simulink model "smd_closedloop"  (R2026a)
settings: Solver=VariableStepAuto  StopTime=12
undefined symbols (not defined in the file): c, k, m
settings Model: Creator=tdxt  LastModifiedBy=tdxt

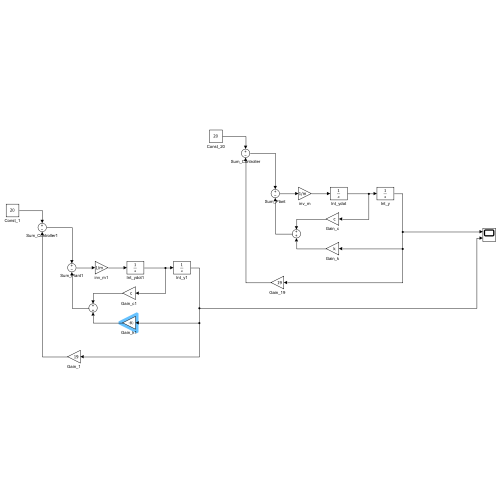
[thumbnail: Simulink's stored preview of the top-level diagram]
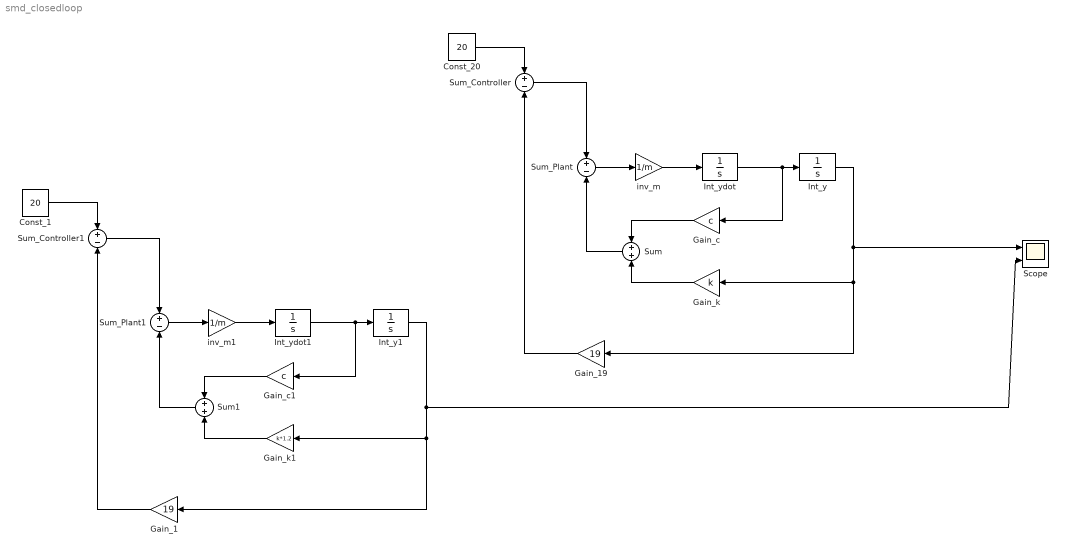
== system smd_closedloop ==
  Const_1 : Constant  Value=20
  Const_20 : Constant  Value=20
  Gain_1 : Gain  Gain=19
  Gain_19 : Gain  Gain=19
  Gain_c : Gain  Gain=c
  Gain_c1 : Gain  Gain=c
  Gain_k : Gain  Gain=k
  Gain_k1 : Gain  Gain=k*1.2
  Int_y : Integrator
  Int_y1 : Integrator
  Int_ydot : Integrator
  Int_ydot1 : Integrator
  Scope : Scope  NumInputPorts=2
      settings: ActiveDisplayYMinimum=0.20136921738041336  ActiveDisplayYMaximum=1.7818905379444292
  Sum : Sum
  Sum1 : Sum
  Sum_Controller : Sum  Inputs=+-
  Sum_Controller1 : Sum  Inputs=+-
  Sum_Plant : Sum  Inputs=+-
  Sum_Plant1 : Sum  Inputs=+-
  inv_m : Gain  Gain=1/m
  inv_m1 : Gain  Gain=1/m
  wires:
  Const_20/1 -> Sum_Controller/1
  Sum_Controller/1 -> Sum_Plant/1
  Sum/1 -> Sum_Plant/2
  Gain_k/1 -> Sum/2
  inv_m/1 -> Int_ydot/1
  Sum_Plant/1 -> inv_m/1
  Gain_19/1 -> Sum_Controller/2
  Gain_c/1 -> Sum/1
  Int_ydot/1 -> Gain_c/1, Int_y/1
  Int_y/1 -> Gain_k/1, Gain_19/1, Scope/1
  Int_y1/1 -> Scope/2, Gain_1/1, Gain_k1/1
  Int_ydot1/1 -> Int_y1/1, Gain_c1/1
  Gain_c1/1 -> Sum1/1
  Gain_1/1 -> Sum_Controller1/2
  Sum_Plant1/1 -> inv_m1/1
  inv_m1/1 -> Int_ydot1/1
  Gain_k1/1 -> Sum1/2
  Sum1/1 -> Sum_Plant1/2
  Sum_Controller1/1 -> Sum_Plant1/1
  Const_1/1 -> Sum_Controller1/1
